simulink model "glucose_model"  (R2022a)
settings: Solver=VariableStepAuto  StartTime=0.0  StopTime=10.0  RelTol=1e-3
undefined symbols (not defined in the file): G, Gb, I, k1, k2
settings Model: Creator=dell  LastModifiedBy=dell

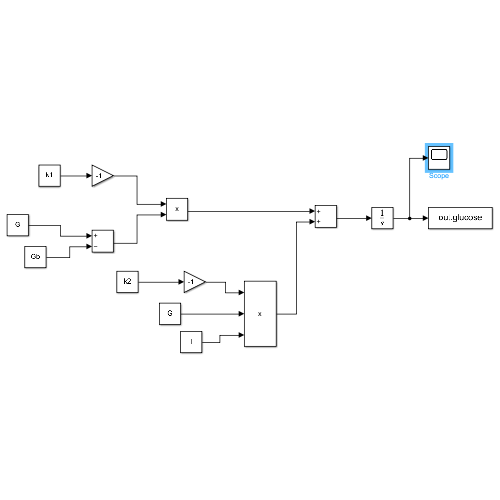
[thumbnail: Simulink's stored preview of the top-level diagram]
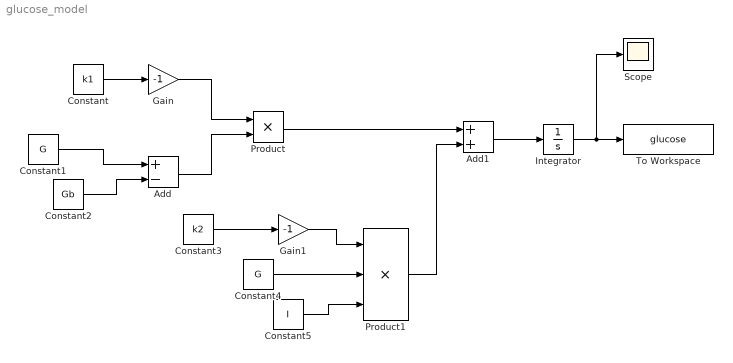
== system glucose_model ==
  Add : Sum  Inputs=+-
  Add1 : Sum
  Constant : Constant  Value=k1
  Constant1 : Constant  Value=G
  Constant2 : Constant  Value=Gb
  Constant3 : Constant  Value=k2
  Constant4 : Constant  Value=G
  Constant5 : Constant  Value=I
  Gain : Gain  Gain=-1
  Gain1 : Gain  Gain=-1
  Integrator : Integrator
  Product : Product
  Product1 : Product  Inputs=3
  Scope : Scope
  To Workspace : ToWorkspace  VariableName=glucose  SaveFormat=Timeseries  SampleTime=-1
  wires:
  Constant/1 -> Gain/1
  Gain/1 -> Product/1
  Constant1/1 -> Add/1
  Constant2/1 -> Add/2
  Add/1 -> Product/2
  Product/1 -> Add1/1
  Constant4/1 -> Product1/2
  Constant5/1 -> Product1/3
  Constant3/1 -> Gain1/1
  Gain1/1 -> Product1/1
  Product1/1 -> Add1/2
  Add1/1 -> Integrator/1
  Integrator/1 -> To Workspace/1, Scope/1
